simulink model "controller"  (R2022b)
settings: Solver=VariableStepAuto  StartTime=0.0  StopTime=5.0  RelTol=1e-3
values from neighbouring files (symbols this model uses):
  dq_10 = 0    [mainScript.m]
  dq_20 = 0    [mainScript.m]
  K0 = diag([K0  K0])    [GSOPD.m]    (also in mainScript.m = 45)
  K1 = diag([K1  K1])    [GSOPD.m]    (also in mainScript.m = 40)
  kd1 = x(13)    [GSOPD.m]    (also in mainScript.m = 33)
  kd2 = x(14)    [GSOPD.m]    (also in mainScript.m = 10)
  kp1 = x(11)    [GSOPD.m]    (also in mainScript.m = 80)
  kp2 = x(12)    [GSOPD.m]    (also in mainScript.m = 100)
  p1 = x(5)    [GSOPD.m]    (also in dynamic_terms.m = robot_parameters(1); mainScript.m = 8.77; open_loop_dynamics.m = x(7))
  p2 = x(6)    [GSOPD.m]    (also in dynamic_terms.m = robot_parameters(2); mainScript.m = 0.51; open_loop_dynamics.m = x(8))
  p3 = x(7)    [GSOPD.m]    (also in dynamic_terms.m = robot_parameters(3); mainScript.m = 0.76; open_loop_dynamics.m = x(9))
  p4 = x(8)    [GSOPD.m]    (also in dynamic_terms.m = robot_parameters(4); mainScript.m = 0.62; open_loop_dynamics.m = x(10))
  p5 = x(9)    [GSOPD.m]    (also in dynamic_terms.m = robot_parameters(5); mainScript.m = 74.48; open_loop_dynamics.m = x(11))
  p6 = x(10)    [GSOPD.m]    (also in dynamic_terms.m = robot_parameters(6); mainScript.m = 6.174; open_loop_dynamics.m = x(12))
  q_10 = 3    [mainScript.m]
  q_20 = -2    [mainScript.m]
  q_d1 = sin(pi*t)    [mainScript.m]
  q_d2 = sin(pi*t)    [mainScript.m]
settings Model: Creator=َAliiPmD  LastModifiedBy=AliiPmD

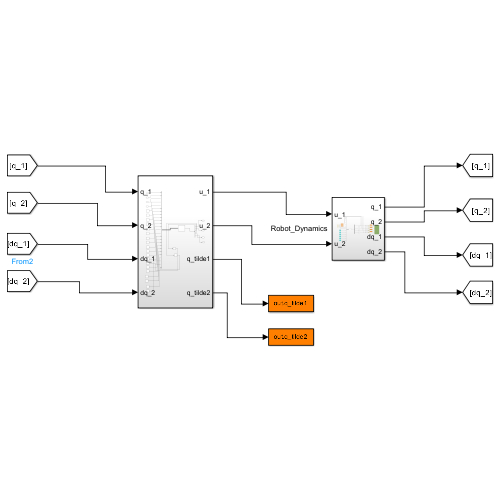
[thumbnail: Simulink's stored preview of the top-level diagram]
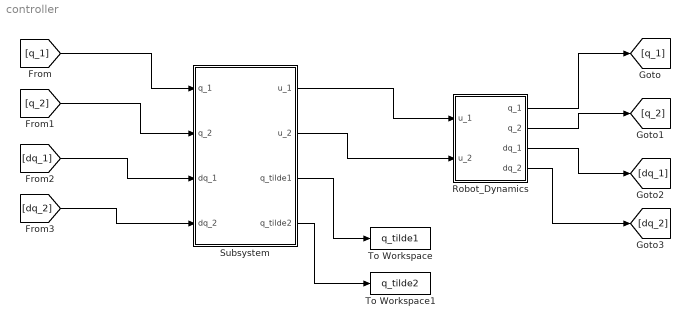
== system controller ==
  Robot_Dynamics : Subsystem
  Subsystem : Subsystem
  To Workspace : ToWorkspace  VariableName=q_tilde1  SampleTime=-1
  To Workspace1 : ToWorkspace  VariableName=q_tilde2  SampleTime=-1
  wires:
  [q_2] -> Subsystem/2(q_2)
  [q_1] -> Subsystem/1(q_1)
  [dq_1] -> Subsystem/3(dq_1)
  [dq_2] -> Subsystem/4(dq_2)
  Subsystem/1(u_1) -> Robot_Dynamics/1(u_1)
  Subsystem/2(u_2) -> Robot_Dynamics/2(u_2)
  Robot_Dynamics/1(q_1) -> [q_1]
  Robot_Dynamics/2(q_2) -> [q_2]
  Robot_Dynamics/3(dq_1) -> [dq_1]
  Robot_Dynamics/4(dq_2) -> [dq_2]
  Subsystem/3(q_tilde1) -> To Workspace/1
  Subsystem/4(q_tilde2) -> To Workspace1/1

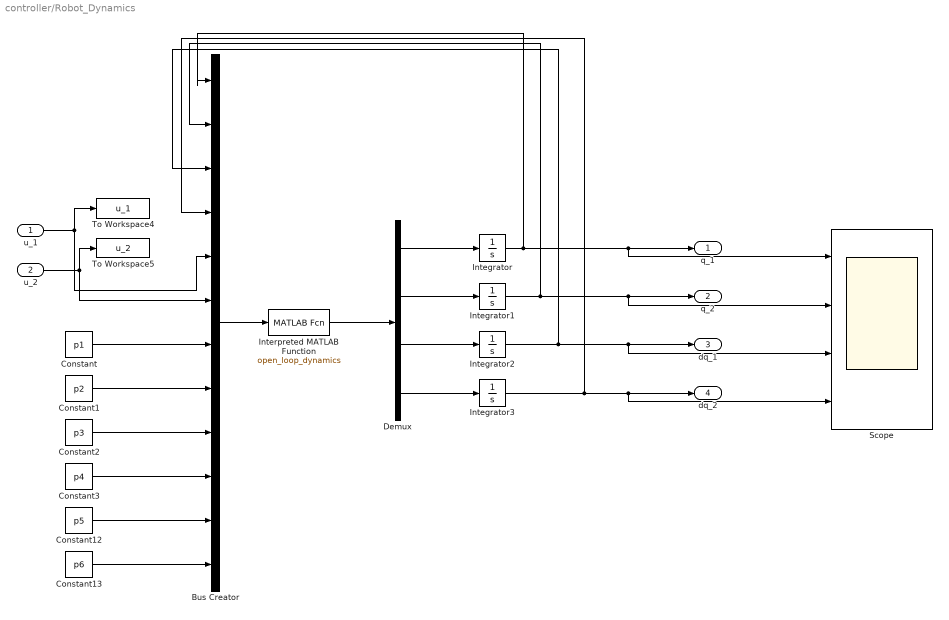
== system controller/Robot_Dynamics ==
  u_1 : Inport
  u_2 : Inport  Port=2
  Bus Creator : BusCreator  Inputs=12
  Constant : Constant  Value=p1
  Constant1 : Constant  Value=p2
  Constant12 : Constant  Value=p5
  Constant13 : Constant  Value=p6
  Constant2 : Constant  Value=p3
  Constant3 : Constant  Value=p4
  Demux : Demux
  Integrator : Integrator  InitialCondition=q_10
  Integrator1 : Integrator  InitialCondition=q_20
  Integrator2 : Integrator  InitialCondition=dq_10
  Integrator3 : Integrator  InitialCondition=dq_20
  Interpreted MATLAB Function : MATLABFcn  MATLABFcn=open_loop_dynamics
  Scope : Scope  NumInputPorts=4
  To Workspace4 : ToWorkspace  VariableName=u_1  SampleTime=-1
  To Workspace5 : ToWorkspace  VariableName=u_2  SampleTime=-1
  q_1 : Outport
  q_2 : Outport  Port=2
  dq_1 : Outport  Port=3
  dq_2 : Outport  Port=4
  wires:
  Integrator1/1 -> Bus Creator/2, q_2/1, Scope/2
  Constant12/1 -> Bus Creator/11
  Integrator2/1 -> Bus Creator/3, dq_1/1, Scope/3
  Constant/1 -> Bus Creator/7
  Constant3/1 -> Bus Creator/10
  Constant13/1 -> Bus Creator/12
  u_1/1 -> Bus Creator/5, To Workspace4/1
  u_2/1 -> Bus Creator/6, To Workspace5/1
  Integrator3/1 -> Bus Creator/4, dq_2/1, Scope/4
  Bus Creator/1 -> Interpreted MATLAB Function/1
  Demux/3 -> Integrator2/1
  Integrator/1 -> q_1/1, Scope/1, Bus Creator/1
  Constant1/1 -> Bus Creator/8
  Constant2/1 -> Bus Creator/9
  Interpreted MATLAB Function/1 -> Demux/1
  Demux/2 -> Integrator1/1
  Demux/4 -> Integrator3/1
  Demux/1 -> Integrator/1

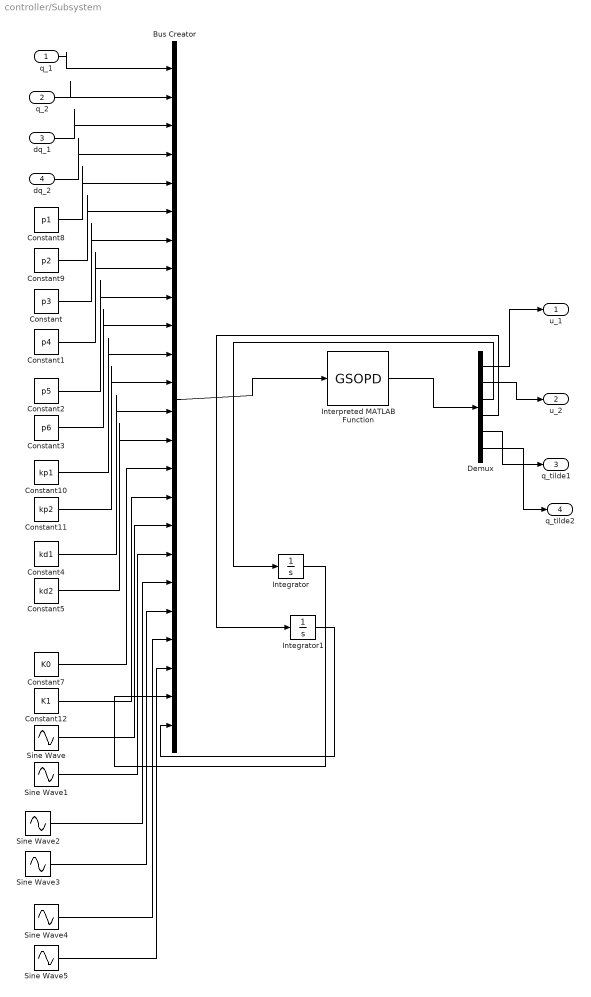
== system controller/Subsystem ==
  q_1 : Inport
  q_2 : Inport  Port=2
  dq_1 : Inport  Port=3
  dq_2 : Inport  Port=4
  Bus Creator : BusCreator  Inputs=24
  Constant : Constant  Value=p3
  Constant1 : Constant  Value=p4
  Constant10 : Constant  Value=kp1
  Constant11 : Constant  Value=kp2
  Constant12 : Constant  Value=K1
  Constant2 : Constant  Value=p5
  Constant3 : Constant  Value=p6
  Constant4 : Constant  Value=kd1
  Constant5 : Constant  Value=kd2
  Constant7 : Constant  Value=K0
  Constant8 : Constant  Value=p1
  Constant9 : Constant  Value=p2
  Demux : Demux  Outputs=6
  Integrator : Integrator  InitialCondition=K0 * (q_10 - q_d1)
  Integrator1 : Integrator  InitialCondition=K0 * (q_20 - q_d2)
  Interpreted MATLAB Function : MATLABFcn  MATLABFcn=GSOPD
  Sine Wave : Sin  Frequency=pi  SampleTime=0
  Sine Wave1 : Sin  Frequency=pi  SampleTime=0
  Sine Wave2 : Sin  Amplitude=pi  Frequency=pi  Phase=pi/2  SampleTime=0
  Sine Wave3 : Sin  Amplitude=pi  Frequency=pi  Phase=pi/2  SampleTime=0
  Sine Wave4 : Sin  Amplitude=-1*pi*pi  Frequency=pi  SampleTime=0
  Sine Wave5 : Sin  Amplitude=-1*pi*pi  Frequency=pi  SampleTime=0
  u_1 : Outport
  u_2 : Outport  Port=2
  q_tilde1 : Outport  Port=3
  q_tilde2 : Outport  Port=4
  wires:
  q_1/1 -> Bus Creator/1
  dq_2/1 -> Bus Creator/4
  Constant8/1 -> Bus Creator/5
  Constant9/1 -> Bus Creator/6
  Constant/1 -> Bus Creator/7
  Constant1/1 -> Bus Creator/8
  Constant2/1 -> Bus Creator/9
  Constant3/1 -> Bus Creator/10
  Constant10/1 -> Bus Creator/11
  Constant11/1 -> Bus Creator/12
  Constant4/1 -> Bus Creator/13
  Constant5/1 -> Bus Creator/14
  Constant7/1 -> Bus Creator/15
  Bus Creator/1 -> Interpreted MATLAB Function/1
  q_2/1 -> Bus Creator/2
  dq_1/1 -> Bus Creator/3
  Demux/1 -> u_1/1
  Demux/2 -> u_2/1
  Interpreted MATLAB Function/1 -> Demux/1
  Constant12/1 -> Bus Creator/16
  Sine Wave/1 -> Bus Creator/17
  Sine Wave1/1 -> Bus Creator/18
  Sine Wave2/1 -> Bus Creator/19
  Sine Wave3/1 -> Bus Creator/20
  Sine Wave4/1 -> Bus Creator/21
  Sine Wave5/1 -> Bus Creator/22
  Integrator/1 -> Bus Creator/23
  Demux/3 -> Integrator/1
  Demux/4 -> Integrator1/1
  Integrator1/1 -> Bus Creator/24
  Demux/5 -> q_tilde1/1
  Demux/6 -> q_tilde2/1
